simulink model "process_smlk"  (R2023b)
settings: Solver=VariableStepAuto  StartTime=0.0  StopTime=100  RelTol=1e-3
settings Model: Creator=djbes  LastModifiedBy=djbes

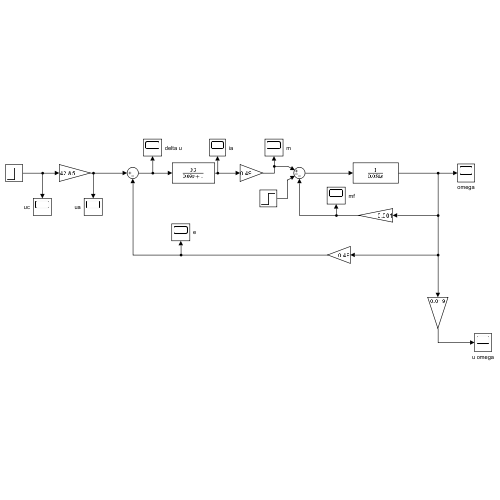
[thumbnail: Simulink's stored preview of the top-level diagram]
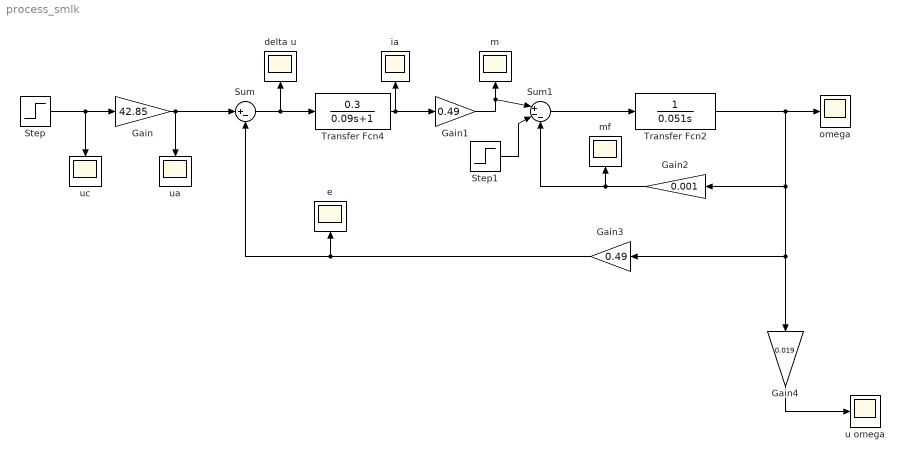
== system process_smlk ==
  Gain : Gain  Gain=42.85
  Gain1 : Gain  Gain=0.49
  Gain2 : Gain  Gain=0.001
  Gain3 : Gain  Gain=0.49
  Gain4 : Gain  Gain=0.019
  Step : Step  After=3.5  SampleTime=0
  Step1 : Step  After=0  SampleTime=0
  Sum : Sum  Inputs=|+-
  Sum1 : Sum  Inputs=|+--
  Transfer Fcn2 : TransferFcn  Denominator=[0.051 0]
  Transfer Fcn4 : TransferFcn  Numerator=[0.3]  Denominator=[0.09 1]
  delta u : Scope
  e : Scope
  ia : Scope
  m : Scope
  mf : Scope
  omega : Scope
  u omega : Scope
  ua : Scope
  uc : Scope
  wires:
  Step/1 -> uc/1, Gain/1
  Gain/1 -> Sum/1, ua/1
  Sum/1 -> Transfer Fcn4/1, delta u/1
  Gain3/1 -> e/1, Sum/2
  Transfer Fcn4/1 -> Gain1/1, ia/1
  Gain1/1 -> Sum1/1, m/1
  Sum1/1 -> Transfer Fcn2/1
  Gain2/1 -> Sum1/3, mf/1
  Transfer Fcn2/1 -> omega/1, Gain4/1, Gain3/1, Gain2/1
  Gain4/1 -> u omega/1
  Step1/1 -> Sum1/2
